simulink model "POMTMRoyerA43333"  (R2021a)
settings: Solver=FixedStepAuto  StartTime=0.0  StopTime=200  FixedStep=1e-4  RelTol=1e-3
settings Model: Creator=mluser  LastModifiedBy=mluser

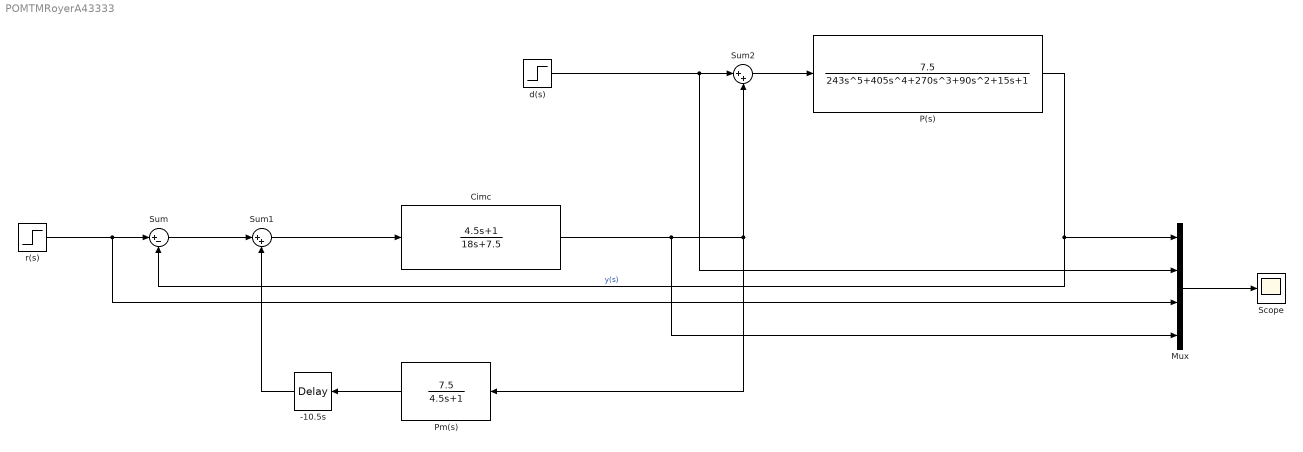
== system POMTMRoyerA43333 ==
  -10.5s : TransportDelay  DelayTime=10.5
  Cimc : TransferFcn  Numerator=[4.5 1]  Denominator=[18 7.5]
  Mux : Mux
  P(s) : TransferFcn  Numerator=[7.5]  Denominator=[243 405 270 90 15 1]
  Pm(s) : TransferFcn  Numerator=[7.5]  Denominator=[4.5 1]
  Scope : Scope
  Sum : Sum  Inputs=|+-
  Sum1 : Sum  Inputs=|++
  Sum2 : Sum  Inputs=|++
  d(s) : Step  Time=80  After=5  SampleTime=0
  r(s) : Step  Time=5  After=15  SampleTime=0
  wires:
  P(s)/1 -> Mux/1, Sum/2  "y(s)"
  r(s)/1 -> Mux/3, Sum/1
  -10.5s/1 -> Sum1/2
  Cimc/1 -> Mux/4, Pm(s)/1, Sum2/2
  Sum/1 -> Sum1/1
  Sum1/1 -> Cimc/1
  d(s)/1 -> Mux/2, Sum2/1
  Pm(s)/1 -> -10.5s/1
  Mux/1 -> Scope/1
  Sum2/1 -> P(s)/1
